simulink model "aptim_refr"  (R2015a)
settings: Solver=ode15s  StartTime=0.0  StopTime=1e4  RelTol=1e-3
values from neighbouring files (symbols this model uses):
  M1 = i/9/2    [optim.m]
libraries: simCryogenics_lib x21, nesl_utility x10
settings Model: Creator=FB229602  LastModifiedBy=FB229602
settings SimscapeCC: SimscapeLogType=all

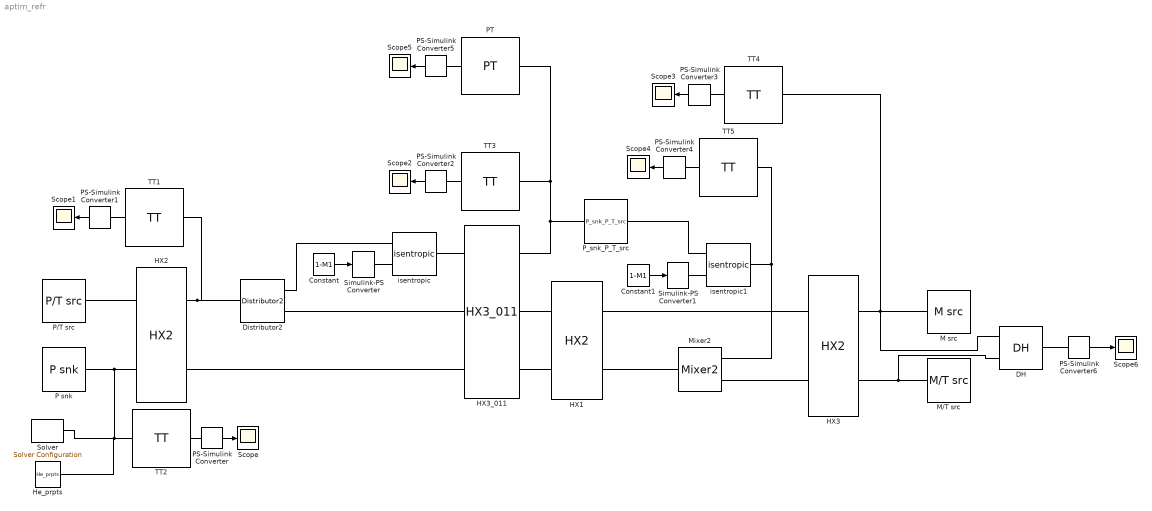
== system aptim_refr ==
  Constant : Constant  Value=1-M1
  Constant1 : Constant  Value=1-M1
  DH : simCryogenics_lib/Sensors/DH
  Distributor2 : simCryogenics_lib/Elements/Distributor2
  HX1 : simCryogenics_lib/Elements/HX2  N=10  Vh=2.3e-3 m^3  Vc=2.3e-3 m^3  M=13 kg  Kh=0 s*bar/kg  Kc=0 s*bar/kg  h=1e4 J/s/K  Th0=300 K  Ph0=16 bar  Mc0=1 kg/s  Tc0=70 K  Pc0=1.05 bar  Mh0=1 kg/s
  HX2 : simCryogenics_lib/Elements/HX2  N=10  Vh=2.3e-3 m^3  Vc=2.3e-3 m^3  M=13 kg  Kh=0 s*bar/kg  Kc=0 s*bar/kg  h=5e4 J/s/K  Th0=300 K  Ph0=16 bar  Mc0=1 kg/s  Tc0=70 K  Pc0=1.05 bar  Mh0=1 kg/s
  HX3 : simCryogenics_lib/Elements/HX2  N=10  Vh=2.3e-3 m^3  Vc=2.3e-3 m^3  M=13 kg  Kh=0 s*bar/kg  Kc=0 s*bar/kg  h=2e4 J/s/K  Th0=300 K  Ph0=16 bar  Mc0=1 kg/s  Tc0=70 K  Pc0=1.05 bar  Mh0=1 kg/s
  HX3_011 : simCryogenics_lib/Elements/HX3_011  N=10  Vh=2.3e-3 m^3  Vm=2.3e-3 m^3  Vc=2.3e-3 m^3  M=13 kg  Kh=0 s*bar/kg  Km=0 s*bar/kg  Kc=0 s*bar/kg  hh_m=2e4 J/s/K  hh_c=2e4 J/s/K  hm_c=2e4 J/s/K  Th0=80 K  Ph0=16 bar  Mh0=0.5 kg/s  Tm0=110 K  Pm0=1.1 bar  Mm0=0.5 kg/s  Tc0=80 K  Pc0=5 bar  Mc0=0.5 kg/s  sensh=0  sensm=1  sensc=1
  He_prpts : simCryogenics_lib/Utilities/He_prpts  P_min=0.1 bar  T_min=5 K  T_max=320 K  P_max=20 bar  Mol=4.0026 * 10 ^ (- 3) kg/mol
  M src : simCryogenics_lib/Sources_Sinks/M src  M=M1 kg/s
  M/T src : simCryogenics_lib/Sources_Sinks/M//T src  M=M1 kg/s  T=4.6 K
  Mixer2 : simCryogenics_lib/Elements/Mixer2
  P snk : simCryogenics_lib/Sources_Sinks/P snk  P=1.05 bar
  P/T src : simCryogenics_lib/Sources_Sinks/P//T src  P=16 bar  T=300 K
  PS-Simulink Converter{,1..6} (7 alike) : nesl_utility/PS-Simulink Converter  PhysicalDomain=network_engine_domain  SubClassName=ps_output  LeftPortType=input  RightPortType=output  PseudoPeriodic=off  Frequencies=[]  Unit=1  AffineConversion=off
  PT : simCryogenics_lib/Sensors/PT
  P_snk_P_T_src : simCryogenics_lib/Sources_Sinks/P_snk_P_T_src  P=5 bar
  Scope{,1..6} (7 alike) : Scope
      Scope1 settings: TimeRange=10  YMin=117.475  YMax=117.5
      Scope2 settings: TimeRange=1000  YMin=117  YMax=122  SaveName=ScopeData2
      Scope3 settings: TimeRange=1000  YMin=9.87  YMax=9.8875  SaveName=Tc
      Scope4 settings: TimeRange=1000  YMin=5.9675  YMax=5.9925  SaveName=ScopeData4
      Scope5 settings: TimeRange=10000  YMin=4  YMax=6  SaveName=ScopeData3
      Scope6 settings: TimeRange=1000  YMin=700  YMax=1500  SaveName=DH
  Simulink-PS Converter : nesl_utility/Simulink-PS Converter  PhysicalDomain=network_engine_domain  SubClassName=ps_input  LeftPortType=input  RightPortType=output  PseudoPeriodic=off  Frequencies=[]  NoiseDistribution=none  NoiseParameters=[]  Unit=1  AffineConversion=off  InputFiltering=off  SimscapeFilterOrder=1  InputFilterTimeConstant=0.001  UdotUserProvided=1
  Simulink-PS Converter1 : nesl_utility/Simulink-PS Converter  PhysicalDomain=network_engine_domain  SubClassName=ps_input  LeftPortType=input  RightPortType=output  PseudoPeriodic=off  Frequencies=[]  NoiseDistribution=none  NoiseParameters=[]  Unit=1  AffineConversion=off  InputFiltering=off  SimscapeFilterOrder=1  InputFilterTimeConstant=0.001  UdotUserProvided=1
  Solver : nesl_utility/Solver Configuration  PhysicalDomain=network_engine_domain  SubClassName=solver  LeftPortType=input  RightPortType=generic  Accelerate=off  Tones=[]  Harmonics=[]  SimulateNoise=off  Profile=off  UseLocalSampling=off  EnableSwitchedLinearOptims=on  FrequencyDomain=off  UseCCode=off  RelTol=0.001  AbsTol=1e-06  MinStep=1e-09  ToWorkspace=off  RevertToSquareIcSolve=off  NumHomotopyIterations=100  DoDC=off  ResidualTolerance=1e-09  UseLocalSolver=off  LocalSolverChoice=NE_BACKWARD_EULER_ADVANCER  LocalSolverSampleTime=0.001  DoFixedCost=off  MaxNonlinIter=3  MaxModeIter=2  LinearAlgebra=Sparse  DelaysMemoryBudget=1024  AutomaticFiltering=on  FilteringTimeConstant=0.001
  TT{1..5} (5 alike) : simCryogenics_lib/Sensors/TT
  isentropic : simCryogenics_lib/Elements/isentropic  eta=0.8  Sin_specify=off  Sin_priority=High  Sin=0 kJ/kg  HoutIs_specify=off  HoutIs_priority=High  HoutIs=0 kJ/kg  Q_specify=off  Q_priority=High  Q=0 W
  isentropic1 : simCryogenics_lib/Elements/isentropic  eta=0.8  Sin_specify=off  Sin_priority=High  Sin=0 kJ/kg  HoutIs_specify=off  HoutIs_priority=High  HoutIs=0 kJ/kg  Q_specify=off  Q_priority=High  Q=0 W
  wires:
  PS-Simulink Converter/1 -> Scope/1
  PS-Simulink Converter1/1 -> Scope1/1
  Constant/1 -> Simulink-PS Converter/1
  Constant1/1 -> Simulink-PS Converter1/1
  PS-Simulink Converter3/1 -> Scope3/1
  PS-Simulink Converter4/1 -> Scope4/1
  PS-Simulink Converter5/1 -> Scope5/1
  PS-Simulink Converter6/1 -> Scope6/1
  PS-Simulink Converter2/1 -> Scope2/1
  connections:
  TT2/LConn1 -- He_prpts/RConn1 -- Solver/RConn1 -- P snk/RConn1 -- HX2/LConn1
  HX2/RConn2 -- Distributor2/LConn1 -- TT1/LConn1
  PS-Simulink Converter/LConn1 -- TT2/RConn1
  PS-Simulink Converter1/LConn1 -- TT1/RConn1
  P/T src/RConn1 -- HX2/LConn2
  isentropic/LConn1 -- Distributor2/RConn1
  Simulink-PS Converter/RConn1 -- isentropic/LConn2
  HX3_011/RConn1 -- isentropic/RConn1
  PS-Simulink Converter2/LConn1 -- TT3/RConn1
  HX3_011/RConn3 -- HX2/RConn1
  HX3_011/RConn2 -- Distributor2/RConn2
  HX1/LConn1 -- HX3_011/LConn3
  HX1/LConn2 -- HX3_011/LConn2
  TT3/LConn1 -- HX3_011/LConn1 -- P_snk_P_T_src/LConn1 -- PT/LConn1
  Simulink-PS Converter1/RConn1 -- isentropic1/LConn2
  P_snk_P_T_src/RConn1 -- isentropic1/LConn1
  isentropic1/RConn1 -- TT5/LConn1 -- Mixer2/LConn2
  HX3/LConn2 -- HX1/RConn2
  PS-Simulink Converter3/LConn1 -- TT4/RConn1
  PS-Simulink Converter4/LConn1 -- TT5/RConn1
  PT/RConn1 -- PS-Simulink Converter5/LConn1
  HX3/RConn2 -- DH/LConn1 -- TT4/LConn1 -- M src/RConn1
  M/T src/RConn1 -- DH/LConn2 -- HX3/RConn1
  Mixer2/RConn1 -- HX1/RConn1
  HX3/LConn1 -- Mixer2/LConn1
  PS-Simulink Converter6/LConn1 -- DH/RConn1
